simulink model "solar_system_model"  (R2024b)
settings: Solver=ode45  StartTime=0.0  StopTime=t_final  MaxStep=3600  RelTol=1e-3
values from neighbouring files (symbols this model uses):
  g = 6.6743e-11    [solar_system.m]
  m = [m_soare, m_mercur, m_venus, m_pamant, m_marte, m_jupiter, m_saturn, m_uranus, m_neptun]    [solar_system.m]
  r0 = zeros(N, 3)    [solar_system.m]
  v0 = zeros(N, 3)    [solar_system.m]
settings Model: Creator=Andreea  LastModifiedBy=Andreea

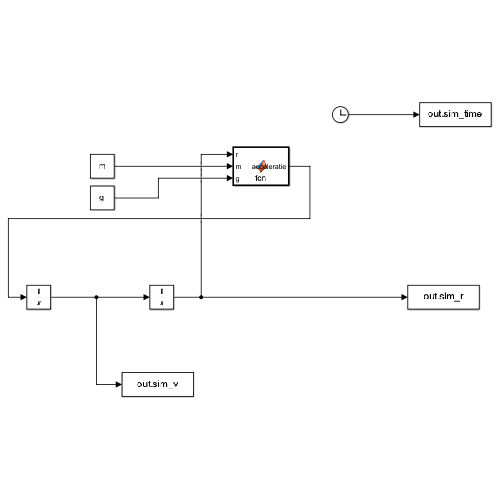
[thumbnail: Simulink's stored preview of the top-level diagram]
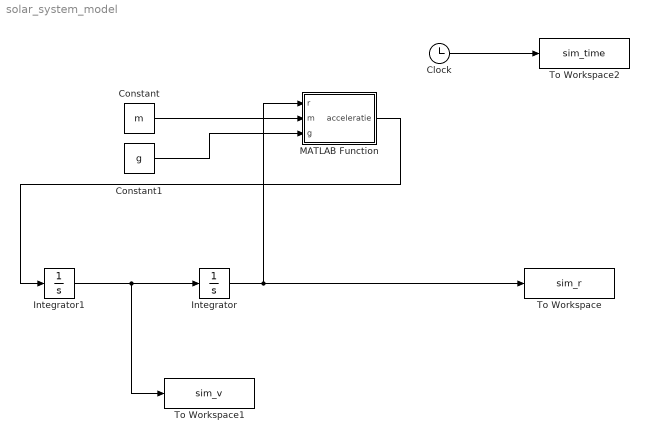
== system solar_system_model ==
  Clock : Clock
  Constant : Constant  Value=m
  Constant1 : Constant  Value=g
  Integrator : Integrator  InitialCondition=r0
  Integrator1 : Integrator  InitialCondition=v0
  MATLAB Function : MATLAB Function  TreatAsAtomicUnit=on
  To Workspace : ToWorkspace  VariableName=sim_r  SampleTime=-1
  To Workspace1 : ToWorkspace  VariableName=sim_v  SampleTime=-1
  To Workspace2 : ToWorkspace  VariableName=sim_time  SaveFormat=Timeseries  SampleTime=-1
  wires:
  Integrator/1 -> MATLAB Function/1(r), To Workspace/1
  Integrator1/1 -> Integrator/1, To Workspace1/1
  Constant/1 -> MATLAB Function/2(m)
  Constant1/1 -> MATLAB Function/3(g)
  MATLAB Function/1(acceleratie) -> Integrator1/1
  Clock/1 -> To Workspace2/1

== matlab function solar_system_model/MATLAB Function ==
  data: r input; acceleratie output; m input; g input
function acceleratie=fcn(r, m, g)
    acceleratie=zeros(9, 3);
    n=9;
    for i=1:n
        for j=1:n
            if i~=j
                rij=r(j,:)-r(i,:);
                dist=norm(rij);
                acceleratie(i,:)=acceleratie(i,:)+g*m(j)*(rij/(dist^3));
            end
        end
    end
end
